simulink model "Encoder_reader_simulink"  (R2025b)
settings: Solver=FixedStepAuto  StartTime=0.0  StopTime=inf  FixedStep=0.01  RelTol=1e-3  EnableMultiTasking=on
libraries: stm32f4xxblockslib x5, stm32g4xxblockslib x4
settings Model: STM32="{\"EncoderBlockForG4\":[{\"ID\":\"untitled:1\"},{\"ID\":\"Lab3_Encoder:1\"},{\"ID\":\"Encoder_reader_simulink:1\"},{\"ID\":\"Encoder_reader_simulink:52\"},{\"ID\":\"Encoder_reader_simulink:53\"},{\"ID\":\"Encoder_reader_simulink:109\"}],\"DigitalPortRead\":[{\"ID\":\"Encoder_reader_simulink:40\"},{\"ID\":\"Encoder_reader_simulink:41\"},{\"ID\":\"Encoder_reader_simulink:116\"},{\"ID\":\"Encoder_reader_simulink:117\"},{\"ID\":\"Encoder_reader_simulink:118\"}]}"  SimulationMode=external  Creator=User  LastModifiedBy=gongk
settings OptimizationCC: DefaultParameterBehavior=Inlined  EnhancedBackFolding=on  PassReuseOutputArgsAs=Individual arguments  ZeroExternalMemoryAtStartup=off  ZeroInternalMemoryAtStartup=off  MaxStackSize=512  OptimizeBlockOrder=speed  DifferentSizesBufferReuse=on  OptimizationCustomize=off  EfficientTunableParamExpr=on
settings DebuggingCC: ParameterTunabilityLossMsg=error
settings HardwareCC: ProdBitPerPointer=32.0  ProdBitPerSizeT=32.0  ProdBitPerPtrDiffT=32.0  ProdLargestAtomicInteger=Long  ProdLargestAtomicFloat=Double  ProdWordSize=32.0  ProdLongLongMode=on  ProdHWDeviceType=ARM Compatible->ARM Cortex-M
settings SFSimCC: MATLABDynamicMemAlloc=off
settings RTWCC: SystemTargetFile=ert.tlc  HardwareBoard=STM32G4xx Based  TemplateMakefile=ert_default_tmf  Toolchain=GNU Tools for ARM Embedded Processors  Description=Embedded Coder
settings CodeAppCC: ForceParamTrailComments=on  IgnoreCustomStorageClasses=off  OperatorAnnotations=on  SimulinkDataObjDesc=on  SFDataObjDesc=on  InsertBlockDesc=on
settings ERTTargetCC: ExtModeTransport=3.0  ExtModeStaticAlloc=on  ExtModeStaticAllocSize=2048.0  ExtModeMexFile=ext_xcp  ExtModeIntrfLevel=Level2 - Open  TargetLangStandard=C99 (ISO)  CodeReplacementLibrary=ARM Cortex-M  SupportContinuousTime=on

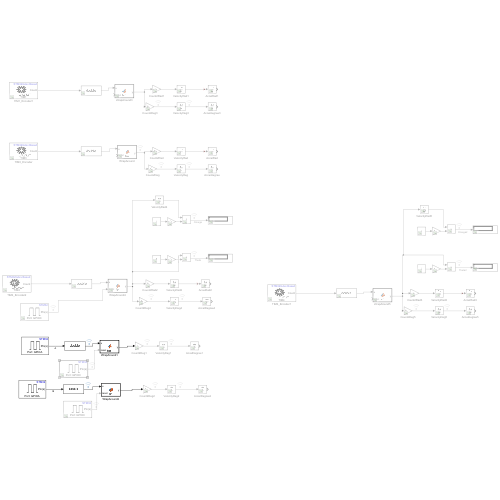
[thumbnail: Simulink's stored preview of the top-level diagram]
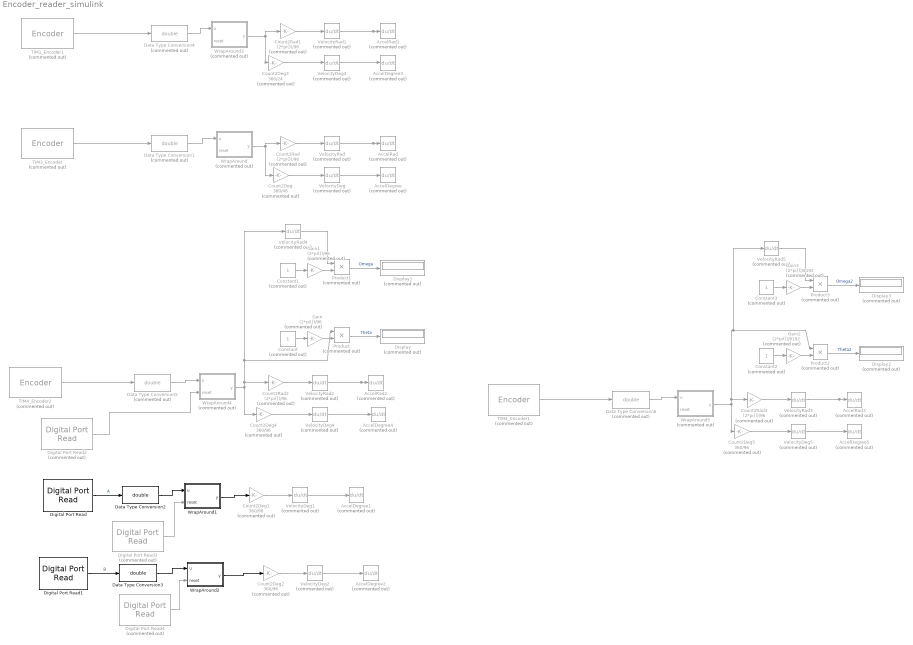
== system Encoder_reader_simulink ==
  AccelDegree{,1..5} (6 alike) : Derivative  Commented=on
  AccelRad{,1..3} (4 alike) : Derivative  Commented=on
  Constant{,1..3} (4 alike) : Constant  Commented=on
  Count2Deg : Gain  Commented=on  Gain=360/48
  Count2Deg{1..2,4..5} (4 alike) : Gain  Commented=on  Gain=360/96
  Count2Deg3 : Gain  Commented=on  Gain=360/24
  Count2Rad{,1..3} (4 alike) : Gain  Commented=on  Gain=(2*pi())/96
  Data Type Conversion{1,4..6} (4 alike) : DataTypeConversion  Commented=on  OutDataTypeStr=double  SaturateOnIntegerOverflow=off  RndMeth=Floor
  Data Type Conversion2 : DataTypeConversion  OutDataTypeStr=double  SaturateOnIntegerOverflow=off  RndMeth=Floor
  Data Type Conversion3 : DataTypeConversion  OutDataTypeStr=double  SaturateOnIntegerOverflow=off  RndMeth=Floor
  Digital Port Read : stm32f4xxblockslib/Digital Port Read  PortName=GPIOA  PinNumber=[4]  ReadOperation=on  IOAsArray=on  SampleTime=-1  EnableSimPort=off  hoistedMaskSrc=ECSoC/ECSimCodegen/Digital Port Read
  Digital Port Read1 : stm32f4xxblockslib/Digital Port Read  PortName=GPIOA  PinNumber=[6]  ReadOperation=on  IOAsArray=on  SampleTime=-1  EnableSimPort=off  hoistedMaskSrc=ECSoC/ECSimCodegen/Digital Port Read
  Digital Port Read2 : stm32f4xxblockslib/Digital Port Read  Commented=on  PortName=GPIOC  PinNumber=[13]  ReadOperation=on  IOAsArray=on  SampleTime=-1  EnableSimPort=off  hoistedMaskSrc=ECSoC/ECSimCodegen/Digital Port Read
      settings: LibrarySourceBlock=stm32g4xxblockslib/Digital Port Read
  Digital Port Read3 : stm32f4xxblockslib/Digital Port Read  Commented=on  PortName=GPIOC  PinNumber=[13]  ReadOperation=on  IOAsArray=on  SampleTime=-1  EnableSimPort=off  hoistedMaskSrc=ECSoC/ECSimCodegen/Digital Port Read
      settings: LibrarySourceBlock=stm32g4xxblockslib/Digital Port Read
  Digital Port Read4 : stm32f4xxblockslib/Digital Port Read  Commented=on  PortName=GPIOC  PinNumber=[13]  ReadOperation=on  IOAsArray=on  SampleTime=-1  EnableSimPort=off  hoistedMaskSrc=ECSoC/ECSimCodegen/Digital Port Read
      settings: LibrarySourceBlock=stm32g4xxblockslib/Digital Port Read
  Display{,1..3} (4 alike) : Display  Commented=on
  Gain : Gain  Commented=on  Gain=(2*pi())/96
  Gain1 : Gain  Commented=on  Gain=(2*pi())/96
  Gain2 : Gain  Commented=on  Gain=(2*pi())/8192
  Gain3 : Gain  Commented=on  Gain=(2*pi())/8192
  Product{,1..3} (4 alike) : Product  Commented=on
  TIM1_Encoder1 : stm32g4xxblockslib/Encoder  Commented=on  TimerModule=TIM1  EnableResetInput=off  OutputCountAfterFirstIndex=off  OutputValidIndex=off  OutputDirection=off  OutputStatus=off  SampleTime=-1
  TIM3_Encoder : stm32g4xxblockslib/Encoder  Commented=on  TimerModule=TIM3  EnableResetInput=off  OutputCountAfterFirstIndex=off  OutputValidIndex=off  OutputDirection=off  OutputStatus=off  SampleTime=-1
  TIM4_Encoder1 : stm32g4xxblockslib/Encoder  Commented=on  TimerModule=TIM4  EnableResetInput=off  OutputCountAfterFirstIndex=off  OutputValidIndex=off  OutputDirection=off  OutputStatus=off  SampleTime=-1
  TIM4_Encoder2 : stm32g4xxblockslib/Encoder  Commented=on  TimerModule=TIM4  EnableResetInput=off  OutputCountAfterFirstIndex=off  OutputValidIndex=off  OutputDirection=off  OutputStatus=off  SampleTime=-1
  VelocityDeg{,1..5} (6 alike) : Derivative  Commented=on
  VelocityRad{,1..5} (6 alike) : Derivative  Commented=on
  WrapAround : MATLAB Function  Commented=on  TreatAsAtomicUnit=on
  WrapAround1 : MATLAB Function  TreatAsAtomicUnit=on
  WrapAround2 : MATLAB Function  TreatAsAtomicUnit=on
  WrapAround3 : MATLAB Function  Commented=on  TreatAsAtomicUnit=on
  WrapAround4 : MATLAB Function  Commented=on  TreatAsAtomicUnit=on
  WrapAround5 : MATLAB Function  Commented=on  TreatAsAtomicUnit=on
  wires:
  TIM3_Encoder/1 -> Data Type Conversion1/1
  Data Type Conversion1/1 -> WrapAround/1(u)
  WrapAround/1(y) -> Count2Rad/1, Count2Deg/1
  Count2Rad/1 -> VelocityRad/1
  Count2Deg/1 -> VelocityDeg/1
  VelocityDeg/1 -> AccelDegree/1
  VelocityRad/1 -> AccelRad/1
  VelocityDeg1/1 -> AccelDegree1/1
  Count2Deg1/1 -> VelocityDeg1/1
  WrapAround1/1(y) -> Count2Deg1/1
  Digital Port Read/1 -> Data Type Conversion2/1  "A"
  Data Type Conversion2/1 -> WrapAround1/1(u)
  Digital Port Read1/1 -> Data Type Conversion3/1  "B"
  Data Type Conversion3/1 -> WrapAround2/1(u)
  WrapAround2/1(y) -> Count2Deg2/1
  VelocityDeg2/1 -> AccelDegree2/1
  Count2Deg2/1 -> VelocityDeg2/1
  VelocityDeg3/1 -> AccelDegree3/1
  VelocityRad1/1 -> AccelRad1/1
  Count2Deg3/1 -> VelocityDeg3/1
  WrapAround3/1(y) -> Count2Rad1/1, Count2Deg3/1
  Count2Rad1/1 -> VelocityRad1/1
  Data Type Conversion4/1 -> WrapAround3/1(u)
  VelocityDeg4/1 -> AccelDegree4/1
  VelocityRad2/1 -> AccelRad2/1
  Count2Deg4/1 -> VelocityDeg4/1
  WrapAround4/1(y) -> VelocityRad4/1, Product/1, Count2Rad2/1, Count2Deg4/1
  Count2Rad2/1 -> VelocityRad2/1
  Data Type Conversion5/1 -> WrapAround4/1(u)
  TIM4_Encoder2/1 -> Data Type Conversion5/1
  TIM1_Encoder1/1 -> Data Type Conversion4/1
  Constant/1 -> Gain/1
  Gain/1 -> Product/2
  Product/1 -> Display/1  "Theta"
  VelocityRad4/1 -> Product1/1
  Gain1/1 -> Product1/2
  Product1/1 -> Display1/1  "Omega"
  Constant1/1 -> Gain1/1
  Constant3/1 -> Gain3/1
  Gain3/1 -> Product3/2
  Product3/1 -> Display3/1  "Omega2"
  VelocityRad5/1 -> Product3/1
  Gain2/1 -> Product2/2
  Product2/1 -> Display2/1  "Theta2"
  Constant2/1 -> Gain2/1
  Count2Rad3/1 -> VelocityRad3/1
  VelocityDeg5/1 -> AccelDegree5/1
  Count2Deg5/1 -> VelocityDeg5/1
  Data Type Conversion6/1 -> WrapAround5/1(u)
  TIM4_Encoder1/1 -> Data Type Conversion6/1
  VelocityRad3/1 -> AccelRad3/1
  WrapAround5/1(y) -> VelocityRad5/1, Product2/1, Count2Rad3/1, Count2Deg5/1
  Digital Port Read2/1 -> WrapAround4/2(reset)
  Digital Port Read3/1 -> WrapAround1/2(reset)
  Digital Port Read4/1 -> WrapAround2/2(reset)

== matlab function Encoder_reader_simulink/WrapAround ==
  data: u input; y output; reset input
function y = fcn(u, reset)

persistent PERIOD;
persistent HALF_PERIOD;
persistent last_raw_count;
persistent accumulated_count;

if isempty(PERIOD)
    PERIOD        = 61440.0;
    HALF_PERIOD   = PERIOD / 2.0; 
end

if isempty(last_raw_count)
    last_raw_count    = u;
    accumulated_count = 0.0;
else
    if reset == 1.0
        accumulated_count = 0.0;
        last_raw_count    = u;
    else
        delta = u - last_raw_count;
        
        if delta < -HALF_PERIOD
            delta = delta + PERIOD; 
            
        elseif delta > HALF_PERIOD
            delta = delta - PERIOD;
        
        end
        
        accumulated_count = accumulated_count + delta;
        last_raw_count = u;
    end
end

y = accumulated_count;
end

== matlab function Encoder_reader_simulink/WrapAround2 ==
  data: u input; y output; reset input
function y = fcn(u, reset)

persistent PERIOD;
persistent HALF_PERIOD;
persistent last_raw_count;
persistent accumulated_count;

if isempty(PERIOD)
    PERIOD        = 61440.0;
    HALF_PERIOD   = PERIOD / 2.0; 
end

if isempty(last_raw_count)
    last_raw_count    = u;
    accumulated_count = 0.0;
else
    if reset == 1.0
        accumulated_count = 0.0;
        last_raw_count    = u;
    else
        delta = u - last_raw_count;
        
        if delta < -HALF_PERIOD
            delta = delta + PERIOD; 
            
        elseif delta > HALF_PERIOD
            delta = delta - PERIOD;
        
        end
        
        accumulated_count = accumulated_count + delta;
        last_raw_count = u;
    end
end

y = accumulated_count;
end

== matlab function Encoder_reader_simulink/WrapAround3 ==
  data: u input; y output; reset input
function y = fcn(u, reset)

persistent PERIOD;
persistent HALF_PERIOD;
persistent last_raw_count;
persistent accumulated_count;

if isempty(PERIOD)
    PERIOD        = 61440.0;
    HALF_PERIOD   = PERIOD / 2.0; 
end

if isempty(last_raw_count)
    last_raw_count    = u;
    accumulated_count = 0.0;
else
    if reset == 1.0
        accumulated_count = 0.0;
        last_raw_count    = u;
    else
        delta = u - last_raw_count;
        
        if delta < -HALF_PERIOD
            delta = delta + PERIOD; 
            
        elseif delta > HALF_PERIOD
            delta = delta - PERIOD;
        
        end
        
        accumulated_count = accumulated_count + delta;
        last_raw_count = u;
    end
end

y = accumulated_count;
end

== matlab function Encoder_reader_simulink/WrapAround4 ==
  data: u input; y output; reset input
function y = fcn(u, reset)

persistent PERIOD;
persistent HALF_PERIOD;
persistent last_raw_count;
persistent accumulated_count;

if isempty(PERIOD)
    PERIOD        = 61440.0;
    HALF_PERIOD   = PERIOD / 2.0; 
end

if isempty(last_raw_count)
    last_raw_count    = u;
    accumulated_count = 0.0;
else
    if reset == 1.0
        accumulated_count = 0.0;
        last_raw_count    = u;
    else
        delta = u - last_raw_count;
        
        if delta < -HALF_PERIOD
            delta = delta + PERIOD; 
            
        elseif delta > HALF_PERIOD
            delta = delta - PERIOD;
        
        end
        
        accumulated_count = accumulated_count + delta;
        last_raw_count = u;
    end
end

y = accumulated_count;
end

== matlab function Encoder_reader_simulink/WrapAround5 ==
  data: u input; y output; reset input
function y = fcn(u, reset)

persistent PERIOD;
persistent HALF_PERIOD;
persistent last_raw_count;
persistent accumulated_count;

if isempty(PERIOD)
    PERIOD        = 61440.0;
    HALF_PERIOD   = PERIOD / 2.0; 
end

if isempty(last_raw_count)
    last_raw_count    = u;
    accumulated_count = 0.0;
else
    if reset == 1.0
        accumulated_count = 0.0;
        last_raw_count    = u;
    else
        delta = u - last_raw_count;
        
        if delta < -HALF_PERIOD
            delta = delta + PERIOD; 
            
        elseif delta > HALF_PERIOD
            delta = delta - PERIOD;
        
        end
        
        accumulated_count = accumulated_count + delta;
        last_raw_count = u;
    end
end

y = accumulated_count;
end

== matlab function Encoder_reader_simulink/WrapAround1 ==
  data: u input; y output; reset input
function y = fcn(u, reset)

persistent PERIOD;
persistent HALF_PERIOD;
persistent last_raw_count;
persistent accumulated_count;

if isempty(PERIOD)
    PERIOD        = 61440.0;
    HALF_PERIOD   = PERIOD / 2.0; 
end

if isempty(last_raw_count)
    last_raw_count    = u;
    accumulated_count = 0.0;
else
    if reset == 1.0
        accumulated_count = 0.0;
        last_raw_count    = u;
    else
        delta = u - last_raw_count;
        
        if delta < -HALF_PERIOD
            delta = delta + PERIOD; 
            
        elseif delta > HALF_PERIOD
            delta = delta - PERIOD;
        
        end
        
        accumulated_count = accumulated_count + delta;
        last_raw_count = u;
    end
end

y = accumulated_count;
end
